simulink model "Final_Project_EEM_EKF_SIM"  (R2020a)
settings: Solver=ode45  StartTime=0  StopTime=t_runtime  FixedStep=clockt/4  RelTol=1e-3  AbsTol=1e-6
PreLoadFcn:
  | run(fullfile('Final_Project_EEM_SIM_init_params.m'));
StopFcn:
  | run('EKF_Simulation_Run_Plots_EEM.m');
values from neighbouring files (symbols this model uses):
  alph1 = Force*L_arm/I1    (= 0.055)    [Final_Project_EEM_SIM_init_params.m]
  alphs1 = 0.1*alph1    (= 0.0055)    [Final_Project_EEM_SIM_init_params.m]
  alphsu = 0.1*alphu    [Final_Project_EEM_SIM_init_params.m]
  alphsv = 0.1*alphv    [Final_Project_EEM_SIM_init_params.m]
  alphu = [sqrt(2) sqrt(2)]/2*[alph2 alph3]'    [Final_Project_EEM_SIM_init_params.m]
  alphv = [-sqrt(2) sqrt(2)]/2*[alph2 alph3]'    [Final_Project_EEM_SIM_init_params.m]
  clockt = 1/200    (= 0.005)    [Final_Project_EEM_SIM_init_params.m]
  DB = 0.345*pi/180    (= 0.00602138591938)    [Final_Project_EEM_SIM_init_params.m]
  delt = .1    (= 0.1)    [Final_Project_EEM_SIM_init_params.m]
  euler_0 = [-30 -10 -60]    [Final_Project_EEM_SIM_init_params.m]
  f_moon = .0012    (= 0.0012)    [Final_Project_EEM_SIM_init_params.m]
  Force = 100    [Final_Project_EEM_SIM_init_params.m]
  Inertia_0 = diag([I2,I3,I1],0)    [Final_Project_EEM_SIM_init_params.m]
  L_arm = 5.5    [Final_Project_EEM_SIM_init_params.m]
  lla_0 = [0.6, 23, 50000]    [Final_Project_EEM_SIM_init_params.m]
  mass_0 = 33296    [Final_Project_EEM_SIM_init_params.m]
  omega_moon = 2.7e-6    (= 2.7e-06)    [Final_Project_EEM_SIM_init_params.m]
  pqr_0 = [0.5730    0.5730    6.8080]    [Final_Project_EEM_SIM_init_params.m]
  r_moon_eq = 5702428    [Final_Project_EEM_SIM_init_params.m]
  tmin = 0.014    [Final_Project_EEM_SIM_init_params.m]
  vel_0 = angle2dcm(euler_0(3)*pi/180, euler_0(2)*pi/180, euler_0(1)*pi/180, 'ZYX')*vel    [Final_Project_EEM_SIM_init_params.m]
undefined symbols (not defined in the file or in its folder): deg, e0_0, e1_0, e2_0, e3_0, Newton, rad, Raphson, s
libraries: sharedtransform x5, sharedutil x5, aerolibtransform2 x4, shared6dofsys x3, aerolibconvert2 x3, vrlib x2, aerolibutil x1, aerolibgravity2 x1, aero_libdap x1
(part 3 of 3)

== matlab function Final_Project_EEM_EKF_SIM/Erin's Extended Kalman Filter ==
  settings: updateMethod=DISCRETE
  data: tclock input; Att_Cmd output; x input size=[2 1]; xhat input size=[2 1]; P input size=[2 2]; Accel_Cmd_X output; alt input; Accel_Cmd_Y output; pitch input; Accel_D input size=[1 1]; x_ecef input; y_ecef input; z_ecef input; Accel_Cmd_Z output; x output; xhat output; P output; y_meas output
%% AE6505 Final Project -- Apollo 11 Final Descent: Extended Kalman Filter
% Use of an EKF to improve estimates of the true altitude and range from 
% unreliable proximity sensor data
% Author: Erin McNeil
% Date: 4-25-2024

function [Att_Cmd,Accel_Cmd_X,Accel_Cmd_Y,Accel_Cmd_Z,x,xhat,P,y_meas] = fcn(tclock,x,xhat,P,alt,pitch, Accel_D,x_ecef,y_ecef,z_ecef)
 
% conversion from ECEF coord to AER
    % Sea of Tranquility (target landing site)
    lat0 = 0.6;
    lon0 = 23.5;
    h0 = 0.0012;

    semimajor_axis = 384000; %km
    eccentricity = 0.0549;

    a  = semimajor_axis;
    e2 = eccentricity^2;
    f = e2 / (1 + sqrt(1 - e2));

    h = h0;
    r = h + a;

    phi = lat0;
    rho = r .* cos(phi);

    lambda = lon0;
    z0 = r .* sin(phi);
    x0 = rho .* cos(lambda);
    y0 = rho .* sin(lambda);

    u = x_ecef - x0;
    v = y_ecef - y0;
    w = z_ecef - z0;

    cosPhi = cos(lat0);
    sinPhi = sin(lat0);
    cosLambda = cos(lon0);
    sinLambda = sin(lon0);

    t     =  cosLambda .* u + sinLambda .* v;
    uEast = -sinLambda .* u + cosLambda .* v;

    wUp    =  cosPhi .* t + sinPhi .* w;
    vNorth = -sinPhi .* t + cosPhi .* w;

    xEast = uEast;
    yNorth = vNorth;
    zUp = wUp;

    deg360 = 2*atan2(0,-1);
    r = hypot(xEast,yNorth);
    slantRange = hypot(r,zUp);
    elevationAngle = atan2(zUp,r);
    azimuthAngle = mod(atan2(xEast,yNorth),deg360);
    

    range_x = sqrt(abs((alt^2)-(slantRange^2))); %260nmi*6076 = 1579760 ft from target

        %% parameter inputs
        g = 5.315; %gravity (ft/sec^2)

        %% noise and covariance matrices
        R = 1000; % Measurement noise covariance
        Q = [200000 0;0 1000]; %process noise

        %% Iterations
        dt = 0.005;
        
        %% Simulation
        altitude = alt; %ft
        Range = range_x; %ft
        
        x = [altitude;Range] + diag(sqrt(Q)*randn);
        
        Noise = 7000;
        deg = 500;
        y_meas = x(1) + (Noise*cos(deg*tclock)*randn);

    %% Start of EKF
    A = [0 1; 0 0];
    H = [1 0];
    
    xhat = [altitude;Range] + diag(sqrt(Q)*randn);
    
    y_comp = xhat(1) + sqrt(R)*randn; %Range (ft)
    
    Pdot = A*P + P*A' + Q;
    P = P + P*dt;

    K = P * H' * inv(H * P * H' + R);  
    xhat = xhat + K * (y_meas - y_comp); 
    P = (eye(2) - K*H)*P*(eye(2) - K*H)' + K*R*K'; 
    
%%    Attitude Commands per Altitude Estimation
        
    if (28000 < xhat(1)) && (xhat(1) < 38887)
        cmd_Roll = 0*(pi/180); %rad
        cmd_Pitch = 0*(pi/180); %rad
        cmd_Yaw = 0*(pi/180); %rad
        Att_Cmd = [-30*(pi/180) -10*(pi/180) -60*(pi/180)] + [cmd_Roll cmd_Pitch cmd_Yaw]; 
    elseif (22000 < xhat(1)) && (xhat(1) < 28000)
        cmd_Roll = 0*(pi/180); %rad
        cmd_Pitch = 15*(pi/180); %rad
        cmd_Yaw = 0*(pi/180); %rad
        Att_Cmd = [-30*(pi/180) 0 -60*(pi/180)] + [cmd_Roll cmd_Pitch cmd_Yaw]; 
    elseif (5000 < xhat(1)) && (xhat(1) < 28000)
        cmd_Roll = 0*(pi/180); %rad
        cmd_Pitch = 35*(pi/180); %rad
        cmd_Yaw = 0*(pi/180); %rad
        Att_Cmd = [-30*(pi/180) 0 -60*(pi/180)] + [cmd_Roll cmd_Pitch cmd_Yaw]; 
    elseif (0 < xhat(1)) && (xhat(1) < 5000)
        cmd_Roll = 0*(pi/180); %rad
        cmd_Pitch = 45*(pi/180); %rad
        cmd_Yaw = 0*(pi/180); %rad
        Att_Cmd = [-30*(pi/180) 0 -60*(pi/180)] + [cmd_Roll cmd_Pitch cmd_Yaw]; 
    else
        cmd_Roll = 0*(pi/180); %rad
        cmd_Pitch = -10*(pi/180); %rad
        cmd_Yaw = 0*(pi/180); %rad
       Att_Cmd = [-30*(pi/180) 0 -60*(pi/180)] + [cmd_Roll cmd_Pitch cmd_Yaw]; 
    end
    
    %% LM Descent Engine
    if 0 < xhat(1) < 38887
        Accel_Cmd_X = 0;
        Accel_Cmd_Y = 0;
        Accel_Cmd_Z = 900;
    else
        Accel_Cmd_X = 0;
        Accel_Cmd_Y = 0;
        Accel_Cmd_Z = 0;
    end

end
